simulink library "lib_fuel_converter"  (Simulink 7.9)
settings: Solver=ode45  SolverMode=SingleTasking  StartTime=0.0  StopTime=10.0  RelTol=1e-3
undefined symbols (not defined in the file or in its folder): acc_mech_eff, acc_mech_pwr, acc_mech_trq, air_cp, amb_tmp, cyc_mph, ex_gas_cp, fc_acc_mass, fc_base_mass, fc_c2i_th_cond, fc_c_init_tmp, fc_cl2h_eff, fc_CO2_to_FUELgps, fc_co_map, fc_co_map_c2h, fc_cold, fc_cold_tmp, fc_cp, fc_ct_trq, fc_eff_scale, fc_emisv, fc_exflow_map, fc_ext_sarea, fc_extmp_map, fc_fuel_den, fc_fuel_lhv, fc_fuel_map, fc_fuel_map_c2h, fc_h2x_th_cond, fc_h_air_flow, fc_h_cp, fc_h_init_tmp, fc_hc_map, fc_hc_map_c2h, fc_hood_emisv, fc_hood_sarea, fc_i2x_th_cond, fc_i_init_tmp, fc_inertia, fc_map_spd, fc_map_trq, fc_max_trq, fc_nn_model_name, fc_nox_map, fc_nox_map_c2h, fc_o2_map, fc_pm_map, fc_pm_map_c2h, fc_pwr_scale, fc_spd_scale, fc_trq_scale, fc_tstat, fc_x_init_tmp, fd_ratio, gb_num_init, gb_ratio, pow, vc_idle_spd, vc_key_on, veh_glider_mass ... (+2)
libraries: lib_fuel_converter x6, lib_etc x4
(part 4 of 4)

== system lib_fuel_converter/configurable subsystems/fuel use and EO emis Neural Network Model/fc temp correct/fc temp correct Variable Correction Factors (Map Based)/NOx factor cold-to-hot ==
  x0 : Inport
  y0 : Inport  Port=2
  Mux : Mux  Inputs=2
  S-function : S-Function  FunctionName=sftable2  Parameters=xindex, yindex, table  EnableBusSupport=off
  table out : Outport  InitialOutput=0
  wires:
  Mux/1 -> S-function/1
  x0/1 -> Mux/1
  S-function/1 -> table out/1
  y0/1 -> Mux/2

== system lib_fuel_converter/configurable subsystems/fuel use and EO emis Neural Network Model/fc temp correct/fc temp correct Variable Correction Factors (Map Based)/PM factor cold-to-hot ==
  x0 : Inport
  y0 : Inport  Port=2
  Mux : Mux  Inputs=2
  S-function : S-Function  FunctionName=sftable2  Parameters=xindex, yindex, table  EnableBusSupport=off
  table out : Outport  InitialOutput=0
  wires:
  Mux/1 -> S-function/1
  x0/1 -> Mux/1
  S-function/1 -> table out/1
  y0/1 -> Mux/2

== system lib_fuel_converter/configurable subsystems/fuel use and EO emis Neural Network Model/fc temp correct/fc temp correct Variable Correction Factors (Map Based)/fuel factor cold-to-hot ==
  x0 : Inport
  y0 : Inport  Port=2
  Mux : Mux  Inputs=2
  S-function : S-Function  FunctionName=sftable2  Parameters=xindex, yindex, table  EnableBusSupport=off
  table out : Outport  InitialOutput=0
  wires:
  Mux/1 -> S-function/1
  x0/1 -> Mux/1
  S-function/1 -> table out/1
  y0/1 -> Mux/2
